simulink model "Copy_of_TenMutantsTemplate"  (R2017b)
settings: Solver=ode3  StartTime=0.0  StopTime=inf  FixedStep=ts  RelTol=0.01  EnableMultiTasking=on
InitFcn:
  | ts=0.0005
  | %ts=100e-6;
StartFcn:
  | close all
StopFcn:
  | % Speed Torque Characterstic
  | 
  | 
  | %figure('Units','pixels', ...
  | %'Color',[1 1 1], ...
  | %'Name','Speed Torque Characterstic',...
  | %'NumberTitle','off',...
  | %'Position',[400 50 470 300], ...
  | %'ToolBar','none');
  | 
  | 
  | 
  | %plot(N_pi,Te_pi)
  | %title('Speed Torque Characterstic')
  | %xlabel('Speed [ RPM ]')
  | %ylabel('Electromagnetic Te_pi [ Nm ] ')
  | %grid on
  | %clear p4 p7 param5 param6 param8 parametres visible voltage
  | 
  | 
  | %clc
values from neighbouring files (symbols this model uses):
  TestOrder = [i]    [ExecuteTestSuite.m]    (also in mutants.m)
undefined symbols (not defined in the file or in its folder): emergency_button2, emergency_buttons, tc_simul, tc_size, temperature, trans1, trans2, trans3, trans4
libraries: simulink x44, powerlib_extras x11
(part 1 of 5)
CloseFcn:
  | close all
settings Model: Creator=srikanth  LastModifiedBy=aarrieta
settings DataIOCC: SaveFormat=Array  SignalLoggingSaveFormat=ModelDataLogs  SaveOutput=off  SaveTime=off  TimeSaveName=t  OutputSaveName=speed,torque,ref
settings OptimizationCC: ExpressionDepthLimit=2147483647  LifeSpan=inf
settings DebuggingCC: UnderspecifiedInitializationDetection=Classic  MergeDetectMultiDrivingBlocksExec=none  ParameterPrecisionLossMsg=none  FcnCallInpInsideContextMsg=warning  StateNameClashWarn=warning  SFUnexpectedBacktrackingDiag=warning  SFNoUnconditionalDefaultTransitionDiag=warning  SFExecutionAtInitializationDiag=none
settings HardwareCC: ProdBitPerPointer=32  ProdBitPerSizeT=32  ProdBitPerPtrDiffT=32  ProdLargestAtomicFloat=None  ProdIntDivRoundTo=Undefined  ProdEndianess=Unspecified  ProdWordSize=32  ProdHWDeviceType=32-bit Generic
settings ModelReferenceCC: PropagateSignalLabelsOutOfModel=off
settings CodeAppCC: StateflowObjectComments=on
settings GRTTargetCC: TargetLangStandard=C89/C90 (ANSI)  GeneratePreprocessorConditionals=Disable all  CombineOutputUpdateFcns=off  GRTInterface=on
settings ConfigComp: CovMetricSettings=dw  CovHtmlReporting=on  CovSaveCumulativeToWorkspaceVar=on  CovSaveSingleToWorkspaceVar=on  CovExternalEMLEnable=off

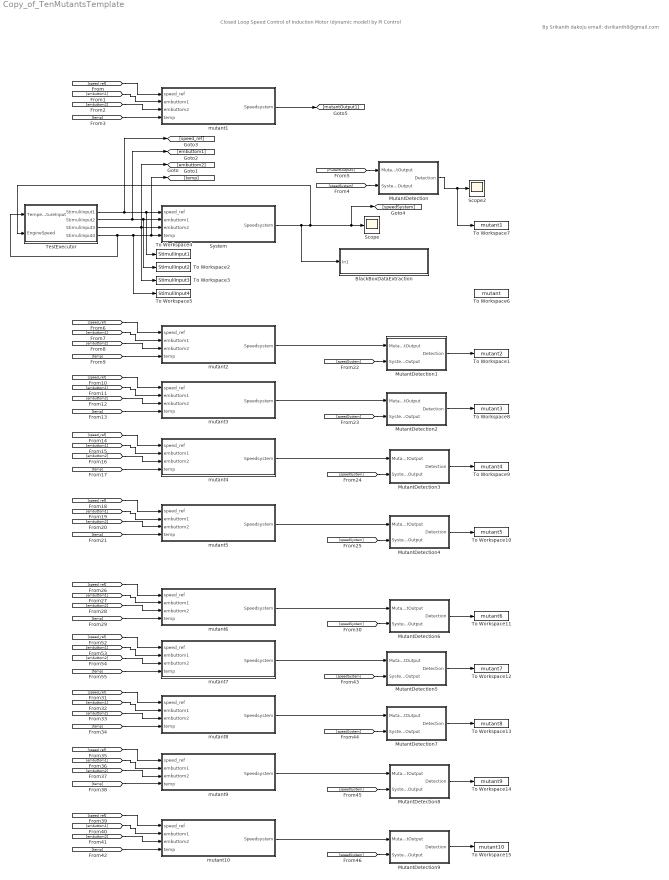
== system Copy_of_TenMutantsTemplate ==
  note: Closed Loop Speed Control of Induction Motor (dynamic model) by PI Control
  note: By
      | Srikanth dakoju
      | email: dsrikanth8@gmail.com
  BlackBoxDataExtraction : Subsystem
  MutantDetection : Subsystem
  MutantDetection1 : Subsystem
  MutantDetection2 : Subsystem
  MutantDetection3 : Subsystem
  MutantDetection4 : Subsystem
  MutantDetection5 : Subsystem
  MutantDetection6 : Subsystem
  MutantDetection7 : Subsystem
  MutantDetection8 : Subsystem
  MutantDetection9 : Subsystem
  Scope : Scope
  Scope2 : Scope
  System : Subsystem
  TestExecutor : Subsystem
  To Workspace1 : ToWorkspace  VariableName=mutant2  SampleTime=-1
  To Workspace10 : ToWorkspace  VariableName=mutant5  SampleTime=-1
  To Workspace11 : ToWorkspace  VariableName=mutant6  SampleTime=-1
  To Workspace12 : ToWorkspace  VariableName=mutant7  SampleTime=-1
  To Workspace13 : ToWorkspace  VariableName=mutant8  SampleTime=-1
  To Workspace14 : ToWorkspace  VariableName=mutant9  SampleTime=-1
  To Workspace15 : ToWorkspace  VariableName=mutant10  SampleTime=-1
  To Workspace2 : ToWorkspace  VariableName=StimuliInput2  SampleTime=-1
  To Workspace3 : ToWorkspace  VariableName=StimuliInput3  SampleTime=-1
  To Workspace4 : ToWorkspace  VariableName=StimuliInput1  SampleTime=-1
  To Workspace5 : ToWorkspace  VariableName=StimuliInput4  SampleTime=-1
  To Workspace6 : ToWorkspace  VariableName=mutant  SampleTime=-1
  To Workspace7 : ToWorkspace  VariableName=mutant1  SampleTime=-1
  To Workspace8 : ToWorkspace  VariableName=mutant3  SampleTime=-1
  To Workspace9 : ToWorkspace  VariableName=mutant4  SampleTime=-1
  mutant1 : Subsystem
  mutant10 : Subsystem
  mutant2 : Subsystem
  mutant3 : Subsystem
  mutant4 : Subsystem
  mutant5 : Subsystem
  mutant6 : Subsystem
  mutant7 : Subsystem
  mutant8 : Subsystem
  mutant9 : Subsystem
  wires:
  TestExecutor/2(StimuliInput2) -> [embuttom1], To Workspace2/1, System/2(embuttom1)
  TestExecutor/3(StimuliInput3) -> [embuttom2], To Workspace3/1, System/3(embuttom2)
  TestExecutor/4(StimuliInput4) -> TestExecutor/1(TemperatureInput), To Workspace5/1, [temp], System/4(temp)
  System/1(Speedsystem) -> BlackBoxDataExtraction/1(In1), TestExecutor/2(EngineSpeed), [speedSystem], Scope/1
  TestExecutor/1(StimuliInput1) -> [speed_ref], To Workspace4/1, System/1(speed_ref)
  mutant1/1(Speedsystem) -> [mutantOutput1]
  MutantDetection/1(Detection) -> To Workspace7/1, Scope2/1
  [temp] -> mutant1/4(temp)
  [embuttom2] -> mutant1/3(embuttom2)
  [embuttom1] -> mutant1/2(embuttom1)
  [speed_ref] -> mutant1/1(speed_ref)
  [speedSystem] -> MutantDetection/2(SystemOutput)
  [mutantOutput1] -> MutantDetection/1(MutantOutput)
  [speed_ref] -> mutant2/1(speed_ref)
  [embuttom1] -> mutant2/2(embuttom1)
  [embuttom2] -> mutant2/3(embuttom2)
  [temp] -> mutant2/4(temp)
  mutant3/1(Speedsystem) -> MutantDetection2/1(MutantOutput)
  [temp] -> mutant3/4(temp)
  [embuttom2] -> mutant3/3(embuttom2)
  [embuttom1] -> mutant3/2(embuttom1)
  [speed_ref] -> mutant3/1(speed_ref)
  [speed_ref] -> mutant4/1(speed_ref)
  [embuttom1] -> mutant4/2(embuttom1)
  [embuttom2] -> mutant4/3(embuttom2)
  [temp] -> mutant4/4(temp)
  mutant5/1(Speedsystem) -> MutantDetection4/1(MutantOutput)
  [temp] -> mutant5/4(temp)
  [embuttom2] -> mutant5/3(embuttom2)
  [embuttom1] -> mutant5/2(embuttom1)
  [speed_ref] -> mutant5/1(speed_ref)
  mutant2/1(Speedsystem) -> MutantDetection1/1(MutantOutput)
  [speedSystem] -> MutantDetection1/2(SystemOutput)
  MutantDetection1/1(Detection) -> To Workspace1/1
  [speedSystem] -> MutantDetection2/2(SystemOutput)
  [speedSystem] -> MutantDetection3/2(SystemOutput)
  mutant4/1(Speedsystem) -> MutantDetection3/1(MutantOutput)
  [speedSystem] -> MutantDetection4/2(SystemOutput)
  MutantDetection4/1(Detection) -> To Workspace10/1
  MutantDetection3/1(Detection) -> To Workspace9/1
  MutantDetection2/1(Detection) -> To Workspace8/1
  MutantDetection6/1(Detection) -> To Workspace11/1
  [speedSystem] -> MutantDetection6/2(SystemOutput)
  [speed_ref] -> mutant6/1(speed_ref)
  [embuttom1] -> mutant6/2(embuttom1)
  [embuttom2] -> mutant6/3(embuttom2)
  [temp] -> mutant6/4(temp)
  mutant6/1(Speedsystem) -> MutantDetection6/1(MutantOutput)
  mutant7/1(Speedsystem) -> MutantDetection5/1(MutantOutput)
  [embuttom1] -> mutant8/2(embuttom1)
  [speed_ref] -> mutant8/1(speed_ref)
  [embuttom2] -> mutant8/3(embuttom2)
  [temp] -> mutant8/4(temp)
  [embuttom1] -> mutant7/2(embuttom1)
  [speed_ref] -> mutant7/1(speed_ref)
  [embuttom2] -> mutant7/3(embuttom2)
  [embuttom2] -> mutant10/3(embuttom2)
  [temp] -> mutant10/4(temp)
  [speed_ref] -> mutant10/1(speed_ref)
  mutant10/1(Speedsystem) -> MutantDetection9/1(MutantOutput)
  mutant8/1(Speedsystem) -> MutantDetection7/1(MutantOutput)
  [speedSystem] -> MutantDetection9/2(SystemOutput)
  [speed_ref] -> mutant9/1(speed_ref)
  [embuttom2] -> mutant9/3(embuttom2)
  [speedSystem] -> MutantDetection7/2(SystemOutput)
  [embuttom1] -> mutant10/2(embuttom1)
  MutantDetection5/1(Detection) -> To Workspace12/1
  mutant9/1(Speedsystem) -> MutantDetection8/1(MutantOutput)
  [temp] -> mutant9/4(temp)
  [embuttom1] -> mutant9/2(embuttom1)
  [speedSystem] -> MutantDetection5/2(SystemOutput)
  [speedSystem] -> MutantDetection8/2(SystemOutput)
  [temp] -> mutant7/4(temp)
  MutantDetection8/1(Detection) -> To Workspace14/1
  MutantDetection7/1(Detection) -> To Workspace13/1
  MutantDetection9/1(Detection) -> To Workspace15/1

== system Copy_of_TenMutantsTemplate/BlackBoxDataExtraction ==
  In1 : Inport
  Abs2 : Abs
  Abs3 : Abs
  Add1 : Sum  Inputs=+-
  Add2 : Sum  Inputs=+-
  Clock : Clock
  Infinite1 : Scope
  Memory{3..7} (5 alike) : Memory
  MinMax2 : MinMax  Function=max  Inputs=2
  MinMax3 : MinMax  Function=max  Inputs=2
  MinMax4 : MinMax  Function=max  Inputs=2
  MinMax5 : MinMax  Inputs=2
  Rate Transition1 : RateTransition
  To Workspace1 : ToWorkspace  VariableName=MaxMin1  SampleTime=-1
  To Workspace10 : ToWorkspace  VariableName=Output1  SampleTime=-1
  To Workspace13 : ToWorkspace  VariableName=Derivative1  SampleTime=-1
  To Workspace14 : ToWorkspace  VariableName=Infinite1  SampleTime=-1
  To Workspace2 : ToWorkspace  VariableName=time  SampleTime=-1
  derive1 : Scope
  throt : Scope
  wires:
  MinMax3/1 -> Memory4/1, To Workspace14/1, Infinite1/1
  Memory3/1 -> MinMax2/2
  MinMax5/1 -> Add2/2, Memory7/1
  Memory7/1 -> MinMax5/2
  Memory4/1 -> MinMax3/2
  MinMax2/1 -> To Workspace13/1, derive1/1, Memory3/1
  MinMax4/1 -> Add2/1, Memory6/1
  Rate Transition1/1 -> MinMax4/1, MinMax5/1, Abs3/1, Add1/1, Memory5/1
  Memory5/1 -> Add1/2
  Abs2/1 -> MinMax2/1
  Abs3/1 -> MinMax3/1
  Add1/1 -> Abs2/1
  Memory6/1 -> MinMax4/2
  Add2/1 -> To Workspace1/1
  In1/1 -> throt/1, Rate Transition1/1, To Workspace10/1
  Clock/1 -> To Workspace2/1

== system Copy_of_TenMutantsTemplate/MutantDetection ==
  MutantOutput : Inport
  SystemOutput : Inport  Port=2
  Logical Operator : Logic  Operator=NOT  AllPortsSameDT=off  OutDataTypeStr=boolean
  Memory : Memory  InitialCondition=1
  MinMax : MinMax  Inputs=2
  Relational Operator : RelationalOperator  Operator===  OutDataTypeStr=boolean  RndMeth=Simplest
  Detection : Outport
  wires:
  Memory/1 -> MinMax/2
  MinMax/1 -> Logical Operator/1, Memory/1
  MutantOutput/1 -> Relational Operator/1
  SystemOutput/1 -> Relational Operator/2
  Relational Operator/1 -> MinMax/1
  Logical Operator/1 -> Detection/1

== system Copy_of_TenMutantsTemplate/MutantDetection1 ==
  MutantOutput : Inport
  SystemOutput : Inport  Port=2
  Logical Operator : Logic  Operator=NOT  AllPortsSameDT=off  OutDataTypeStr=boolean
  Memory : Memory  InitialCondition=1
  MinMax : MinMax  Inputs=2
  Relational Operator : RelationalOperator  Operator===  OutDataTypeStr=boolean  RndMeth=Simplest
  Detection : Outport
  wires:
  Logical Operator/1 -> Detection/1
  Relational Operator/1 -> MinMax/1
  SystemOutput/1 -> Relational Operator/2
  MutantOutput/1 -> Relational Operator/1
  MinMax/1 -> Memory/1, Logical Operator/1
  Memory/1 -> MinMax/2

== system Copy_of_TenMutantsTemplate/MutantDetection2 ==
  MutantOutput : Inport
  SystemOutput : Inport  Port=2
  Logical Operator : Logic  Operator=NOT  AllPortsSameDT=off  OutDataTypeStr=boolean
  Memory : Memory  InitialCondition=1
  MinMax : MinMax  Inputs=2
  Relational Operator : RelationalOperator  Operator===  OutDataTypeStr=boolean  RndMeth=Simplest
  Detection : Outport
  wires:
  Memory/1 -> MinMax/2
  MinMax/1 -> Logical Operator/1, Memory/1
  MutantOutput/1 -> Relational Operator/1
  SystemOutput/1 -> Relational Operator/2
  Relational Operator/1 -> MinMax/1
  Logical Operator/1 -> Detection/1

== system Copy_of_TenMutantsTemplate/MutantDetection3 ==
  MutantOutput : Inport
  SystemOutput : Inport  Port=2
  Logical Operator : Logic  Operator=NOT  AllPortsSameDT=off  OutDataTypeStr=boolean
  Memory : Memory  InitialCondition=1
  MinMax : MinMax  Inputs=2
  Relational Operator : RelationalOperator  Operator===  OutDataTypeStr=boolean  RndMeth=Simplest
  Detection : Outport
  wires:
  Logical Operator/1 -> Detection/1
  Relational Operator/1 -> MinMax/1
  SystemOutput/1 -> Relational Operator/2
  MutantOutput/1 -> Relational Operator/1
  MinMax/1 -> Memory/1, Logical Operator/1
  Memory/1 -> MinMax/2

== system Copy_of_TenMutantsTemplate/MutantDetection4 ==
  MutantOutput : Inport
  SystemOutput : Inport  Port=2
  Logical Operator : Logic  Operator=NOT  AllPortsSameDT=off  OutDataTypeStr=boolean
  Memory : Memory  InitialCondition=1
  MinMax : MinMax  Inputs=2
  Relational Operator : RelationalOperator  Operator===  OutDataTypeStr=boolean  RndMeth=Simplest
  Detection : Outport
  wires:
  Memory/1 -> MinMax/2
  MinMax/1 -> Logical Operator/1, Memory/1
  MutantOutput/1 -> Relational Operator/1
  SystemOutput/1 -> Relational Operator/2
  Relational Operator/1 -> MinMax/1
  Logical Operator/1 -> Detection/1

== system Copy_of_TenMutantsTemplate/MutantDetection5 ==
  MutantOutput : Inport
  SystemOutput : Inport  Port=2
  Logical Operator : Logic  Operator=NOT  AllPortsSameDT=off  OutDataTypeStr=boolean
  Memory : Memory  InitialCondition=1
  MinMax : MinMax  Inputs=2
  Relational Operator : RelationalOperator  Operator===  OutDataTypeStr=boolean  RndMeth=Simplest
  Detection : Outport
  wires:
  Logical Operator/1 -> Detection/1
  Relational Operator/1 -> MinMax/1
  SystemOutput/1 -> Relational Operator/2
  MutantOutput/1 -> Relational Operator/1
  MinMax/1 -> Memory/1, Logical Operator/1
  Memory/1 -> MinMax/2

== system Copy_of_TenMutantsTemplate/MutantDetection6 ==
  MutantOutput : Inport
  SystemOutput : Inport  Port=2
  Logical Operator : Logic  Operator=NOT  AllPortsSameDT=off  OutDataTypeStr=boolean
  Memory : Memory  InitialCondition=1
  MinMax : MinMax  Inputs=2
  Relational Operator : RelationalOperator  Operator===  OutDataTypeStr=boolean  RndMeth=Simplest
  Detection : Outport
  wires:
  Logical Operator/1 -> Detection/1
  Relational Operator/1 -> MinMax/1
  SystemOutput/1 -> Relational Operator/2
  MutantOutput/1 -> Relational Operator/1
  MinMax/1 -> Memory/1, Logical Operator/1
  Memory/1 -> MinMax/2

== system Copy_of_TenMutantsTemplate/MutantDetection7 ==
  MutantOutput : Inport
  SystemOutput : Inport  Port=2
  Logical Operator : Logic  Operator=NOT  AllPortsSameDT=off  OutDataTypeStr=boolean
  Memory : Memory  InitialCondition=1
  MinMax : MinMax  Inputs=2
  Relational Operator : RelationalOperator  Operator===  OutDataTypeStr=boolean  RndMeth=Simplest
  Detection : Outport
  wires:
  Memory/1 -> MinMax/2
  MinMax/1 -> Logical Operator/1, Memory/1
  MutantOutput/1 -> Relational Operator/1
  SystemOutput/1 -> Relational Operator/2
  Relational Operator/1 -> MinMax/1
  Logical Operator/1 -> Detection/1

== system Copy_of_TenMutantsTemplate/MutantDetection8 ==
  MutantOutput : Inport
  SystemOutput : Inport  Port=2
  Logical Operator : Logic  Operator=NOT  AllPortsSameDT=off  OutDataTypeStr=boolean
  Memory : Memory  InitialCondition=1
  MinMax : MinMax  Inputs=2
  Relational Operator : RelationalOperator  Operator===  OutDataTypeStr=boolean  RndMeth=Simplest
  Detection : Outport
  wires:
  Logical Operator/1 -> Detection/1
  Relational Operator/1 -> MinMax/1
  SystemOutput/1 -> Relational Operator/2
  MutantOutput/1 -> Relational Operator/1
  MinMax/1 -> Memory/1, Logical Operator/1
  Memory/1 -> MinMax/2

== system Copy_of_TenMutantsTemplate/MutantDetection9 ==
  MutantOutput : Inport
  SystemOutput : Inport  Port=2
  Logical Operator : Logic  Operator=NOT  AllPortsSameDT=off  OutDataTypeStr=boolean
  Memory : Memory  InitialCondition=1
  MinMax : MinMax  Inputs=2
  Relational Operator : RelationalOperator  Operator===  OutDataTypeStr=boolean  RndMeth=Simplest
  Detection : Outport
  wires:
  Memory/1 -> MinMax/2
  MinMax/1 -> Logical Operator/1, Memory/1
  MutantOutput/1 -> Relational Operator/1
  SystemOutput/1 -> Relational Operator/2
  Relational Operator/1 -> MinMax/1
  Logical Operator/1 -> Detection/1

== system Copy_of_TenMutantsTemplate/System ==
  note: ctrl+U to look under mask
  speed_ref : Inport
  embuttom1 : Inport  Port=2
  embuttom2 : Inport  Port=3
  temp : Inport  Port=4
  "1 HP , 220 V Induction Motor" : Subsystem  mask(Induction Motor: By SRIKANTH D){Rs=10.1, Ls=(15.81+245.8954)/(2*pi*50), Rr=9.8546, Lr=(15.81+245.8954)/(2*pi*50), Lm=(245.8954)/(2*pi*50), J=0.0088, P=4}
      mask prompts: Rs "Stator Resistance  Rs [ohms] :"; Ls "Stator Inductance Ls [Hendry] :"; Rr "Rotor Resistance Rr [ohms] :"; Lr "Rotor Inductance Lr [Hendry] :"; Lm "Mutual Inductance Lm [Hendry] :"; J "Rotor Inertia J [Kg-m2] :"; P "Number of Poles p :"
      mask help: Dynamic Modelling of Induction by using Mathematic Equations
      mask Display: fprintf('Induction\nMotor')
  Data Acquision : Subsystem
  PI Control1 : Subsystem
      mask Display: fprintf('PI\Control')
  Selector : Selector  InputPortWidth=2  IndexOptions=Index vector (dialog)  Indices=[1]  OutputSizes=1
  Subsystem : Subsystem
  Terminator : Terminator
  Terminator1 : Terminator
  VSI : Subsystem
      mask init:
      | Vdc=220;
      mask Display: fprintf('Vdc = 220 V ')
  torque : Step  Time=2  After=0  SampleTime=0
  Speedsystem : Outport
  wires:
  temp/1 -> Subsystem/4(Temperature)
  "1 HP , 220 V Induction Motor"/1(m) -> Data Acquision/1(m)
  VSI/2(Vb) -> "1 HP , 220 V Induction Motor"/3(V_b)
  Data Acquision/3(wm) -> Selector/1  "Speed( rpm)"
  Data Acquision/4(wm1) -> Speedsystem/1
  embuttom2/1 -> Subsystem/3(EmergButton2)
  embuttom1/1 -> Subsystem/2(EmergButton1)
  speed_ref/1 -> Subsystem/1(Speed)
  Data Acquision/2(Te(Nm)) -> Terminator/1  "Torque Te(Nm)"
  Subsystem/1("MotorSpeed ") -> Data Acquision/2(speed), PI Control1/1(N*)
  PI Control1/1(Freq*) -> VSI/1(Freq)
  torque/1 -> "1 HP , 220 V Induction Motor"/1(tau)
  Selector/1 -> PI Control1/2(N)
  VSI/1(Va) -> "1 HP , 220 V Induction Motor"/2(V_a)
  VSI/3(Vc) -> "1 HP , 220 V Induction Motor"/4(V_c)
  Data Acquision/1(is_a) -> Terminator1/1

== system Copy_of_TenMutantsTemplate/TestExecutor ==
  TemperatureInput : Inport
  EngineSpeed : Inport  Port=2
  Constant : Constant  Value=TestOrder
  Constant10 : Constant  Value=trans4
  Constant3 : Constant  Value=tc_simul
  Constant4 : Constant  Value=tc_size
  Constant7 : Constant  Value=trans1
  Constant8 : Constant  Value=trans2
  Constant9 : Constant  Value=trans3
  MATLAB Function : MATLAB Function  TreatAsAtomicUnit=on
  MATLAB Function1 : MATLAB Function  TreatAsAtomicUnit=on
  Memory{,1..3} (4 alike) : Memory  InitialCondition=1
  Scope : Scope
  Scope1 : Scope
  Stop Simulation : Stop
  StimuliInput1 : Outport
  StimuliInput2 : Outport  Port=2
  StimuliInput3 : Outport  Port=3
  StimuliInput4 : Outport  Port=4
  wires:
  Memory3/1 -> MATLAB Function1/7(v_engine)
  Memory2/1 -> MATLAB Function1/8(temp)
  MATLAB Function1/5(simulation_stop) -> Stop Simulation/1
  MATLAB Function1/2(state) -> Scope1/1, MATLAB Function/3(state)
  MATLAB Function1/1(test_case) -> MATLAB Function/2(test_case), Scope/1
  EngineSpeed/1 -> Memory3/1
  Memory1/1 -> MATLAB Function1/9(test_order_id)
  Memory/1 -> MATLAB Function1/10(state_id)
  MATLAB Function1/3(test_order_id1) -> Memory1/1
  MATLAB Function1/4(state_id1) -> Memory/1
  Constant10/1 -> MATLAB Function1/6(trans4)
  Constant9/1 -> MATLAB Function1/5(trans3)
  Constant8/1 -> MATLAB Function1/4(trans2)
  Constant7/1 -> MATLAB Function1/3(trans1)
  Constant4/1 -> MATLAB Function1/2(tc_size)
  Constant/1 -> MATLAB Function1/1(test_order)
  Constant3/1 -> MATLAB Function/1(tc_simul)
  MATLAB Function/4(port_4) -> StimuliInput4/1
  MATLAB Function/3(port_3) -> StimuliInput3/1
  MATLAB Function/2(port_2) -> StimuliInput2/1
  MATLAB Function/1(port_1) -> StimuliInput1/1
  TemperatureInput/1 -> Memory2/1

== system Copy_of_TenMutantsTemplate/mutant1 ==
  note: ctrl+U to look under mask
  speed_ref : Inport
  embuttom1 : Inport  Port=2
  embuttom2 : Inport  Port=3
  temp : Inport  Port=4
  "1 HP , 220 V Induction Motor" : Subsystem  mask(Induction Motor: By SRIKANTH D){Rs=10.1, Ls=(15.81+245.8954)/(2*pi*50), Rr=9.8546, Lr=(15.81+245.8954)/(2*pi*50), Lm=(245.8954)/(2*pi*50), J=0.0088, P=4}
      mask prompts: Rs "Stator Resistance  Rs [ohms] :"; Ls "Stator Inductance Ls [Hendry] :"; Rr "Rotor Resistance Rr [ohms] :"; Lr "Rotor Inductance Lr [Hendry] :"; Lm "Mutual Inductance Lm [Hendry] :"; J "Rotor Inertia J [Kg-m2] :"; P "Number of Poles p :"
      mask help: Dynamic Modelling of Induction by using Mathematic Equations
      mask Display: fprintf('Induction\nMotor')
  Data Acquision : Subsystem
  PI Control1 : Subsystem
      mask Display: fprintf('PI\Control')
  Selector : Selector  InputPortWidth=2  IndexOptions=Index vector (dialog)  Indices=[1]  OutputSizes=1
  Subsystem : Subsystem
  Terminator : Terminator
  Terminator1 : Terminator
  VSI : Subsystem
      mask init:
      | Vdc=220;
      mask Display: fprintf('Vdc = 220 V ')
  torque : Step  Time=2  After=0  SampleTime=0
  Speedsystem : Outport
  wires:
  Data Acquision/1(is_a) -> Terminator1/1
  VSI/3(Vc) -> "1 HP , 220 V Induction Motor"/4(V_c)
  VSI/1(Va) -> "1 HP , 220 V Induction Motor"/2(V_a)
  Selector/1 -> PI Control1/2(N)
  torque/1 -> "1 HP , 220 V Induction Motor"/1(tau)
  PI Control1/1(Freq*) -> VSI/1(Freq)
  Subsystem/1("MotorSpeed ") -> PI Control1/1(N*), Data Acquision/2(speed)
  Data Acquision/2(Te(Nm)) -> Terminator/1  "Torque Te(Nm)"
  speed_ref/1 -> Subsystem/1(Speed)
  embuttom1/1 -> Subsystem/2(EmergButton1)
  embuttom2/1 -> Subsystem/3(EmergButton2)
  Data Acquision/4(wm1) -> Speedsystem/1
  Data Acquision/3(wm) -> Selector/1  "Speed( rpm)"
  VSI/2(Vb) -> "1 HP , 220 V Induction Motor"/3(V_b)
  "1 HP , 220 V Induction Motor"/1(m) -> Data Acquision/1(m)
  temp/1 -> Subsystem/4(Temperature)

== system Copy_of_TenMutantsTemplate/mutant10 ==
  note: ctrl+U to look under mask
  speed_ref : Inport
  embuttom1 : Inport  Port=2
  embuttom2 : Inport  Port=3
  temp : Inport  Port=4
  "1 HP , 220 V Induction Motor" : Subsystem  mask(Induction Motor: By SRIKANTH D){Rs=10.1, Ls=(15.81+245.8954)/(2*pi*50), Rr=9.8546, Lr=(15.81+245.8954)/(2*pi*50), Lm=(245.8954)/(2*pi*50), J=0.0088, P=4}
      mask prompts: Rs "Stator Resistance  Rs [ohms] :"; Ls "Stator Inductance Ls [Hendry] :"; Rr "Rotor Resistance Rr [ohms] :"; Lr "Rotor Inductance Lr [Hendry] :"; Lm "Mutual Inductance Lm [Hendry] :"; J "Rotor Inertia J [Kg-m2] :"; P "Number of Poles p :"
      mask help: Dynamic Modelling of Induction by using Mathematic Equations
      mask Display: fprintf('Induction\nMotor')
  Data Acquision : Subsystem
  PI Control1 : Subsystem
      mask Display: fprintf('PI\Control')
  Selector : Selector  InputPortWidth=2  IndexOptions=Index vector (dialog)  Indices=[1]  OutputSizes=1
  Subsystem : Subsystem
  Terminator : Terminator
  Terminator1 : Terminator
  VSI : Subsystem
      mask init:
      | Vdc=220;
      mask Display: fprintf('Vdc = 220 V ')
  torque : Step  Time=2  After=0  SampleTime=0
  Speedsystem : Outport
  wires:
  Data Acquision/1(is_a) -> Terminator1/1
  VSI/3(Vc) -> "1 HP , 220 V Induction Motor"/4(V_c)
  VSI/1(Va) -> "1 HP , 220 V Induction Motor"/2(V_a)
  Selector/1 -> PI Control1/2(N)
  torque/1 -> "1 HP , 220 V Induction Motor"/1(tau)
  PI Control1/1(Freq*) -> VSI/1(Freq)
  Subsystem/1("MotorSpeed ") -> PI Control1/1(N*), Data Acquision/2(speed)
  Data Acquision/2(Te(Nm)) -> Terminator/1  "Torque Te(Nm)"
  speed_ref/1 -> Subsystem/1(Speed)
  embuttom1/1 -> Subsystem/2(EmergButton1)
  embuttom2/1 -> Subsystem/3(EmergButton2)
  Data Acquision/4(wm1) -> Speedsystem/1
  Data Acquision/3(wm) -> Selector/1  "Speed( rpm)"
  VSI/2(Vb) -> "1 HP , 220 V Induction Motor"/3(V_b)
  "1 HP , 220 V Induction Motor"/1(m) -> Data Acquision/1(m)
  temp/1 -> Subsystem/4(Temperature)

== system Copy_of_TenMutantsTemplate/mutant2 ==
  note: ctrl+U to look under mask
  speed_ref : Inport
  embuttom1 : Inport  Port=2
  embuttom2 : Inport  Port=3
  temp : Inport  Port=4
  "1 HP , 220 V Induction Motor" : Subsystem  mask(Induction Motor: By SRIKANTH D){Rs=10.1, Ls=(15.81+245.8954)/(2*pi*50), Rr=9.8546, Lr=(15.81+245.8954)/(2*pi*50), Lm=(245.8954)/(2*pi*50), J=0.0088, P=4}
      mask prompts: Rs "Stator Resistance  Rs [ohms] :"; Ls "Stator Inductance Ls [Hendry] :"; Rr "Rotor Resistance Rr [ohms] :"; Lr "Rotor Inductance Lr [Hendry] :"; Lm "Mutual Inductance Lm [Hendry] :"; J "Rotor Inertia J [Kg-m2] :"; P "Number of Poles p :"
      mask help: Dynamic Modelling of Induction by using Mathematic Equations
      mask Display: fprintf('Induction\nMotor')
  Data Acquision : Subsystem
  PI Control1 : Subsystem
      mask Display: fprintf('PI\Control')
  Selector : Selector  InputPortWidth=2  IndexOptions=Index vector (dialog)  Indices=[1]  OutputSizes=1
  Subsystem : Subsystem
  Terminator : Terminator
  Terminator1 : Terminator
  VSI : Subsystem
      mask init:
      | Vdc=220;
      mask Display: fprintf('Vdc = 220 V ')
  torque : Step  Time=2  After=0  SampleTime=0
  Speedsystem : Outport
  wires:
  temp/1 -> Subsystem/4(Temperature)
  "1 HP , 220 V Induction Motor"/1(m) -> Data Acquision/1(m)
  VSI/2(Vb) -> "1 HP , 220 V Induction Motor"/3(V_b)
  Data Acquision/3(wm) -> Selector/1  "Speed( rpm)"
  Data Acquision/4(wm1) -> Speedsystem/1
  embuttom2/1 -> Subsystem/3(EmergButton2)
  embuttom1/1 -> Subsystem/2(EmergButton1)
  speed_ref/1 -> Subsystem/1(Speed)
  Data Acquision/2(Te(Nm)) -> Terminator/1  "Torque Te(Nm)"
  Subsystem/1("MotorSpeed ") -> Data Acquision/2(speed), PI Control1/1(N*)
  PI Control1/1(Freq*) -> VSI/1(Freq)
  torque/1 -> "1 HP , 220 V Induction Motor"/1(tau)
  Selector/1 -> PI Control1/2(N)
  VSI/1(Va) -> "1 HP , 220 V Induction Motor"/2(V_a)
  VSI/3(Vc) -> "1 HP , 220 V Induction Motor"/4(V_c)
  Data Acquision/1(is_a) -> Terminator1/1

== system Copy_of_TenMutantsTemplate/mutant3 ==
  note: ctrl+U to look under mask
  speed_ref : Inport
  embuttom1 : Inport  Port=2
  embuttom2 : Inport  Port=3
  temp : Inport  Port=4
  "1 HP , 220 V Induction Motor" : Subsystem  mask(Induction Motor: By SRIKANTH D){Rs=10.1, Ls=(15.81+245.8954)/(2*pi*50), Rr=9.8546, Lr=(15.81+245.8954)/(2*pi*50), Lm=(245.8954)/(2*pi*50), J=0.0088, P=4}
      mask prompts: Rs "Stator Resistance  Rs [ohms] :"; Ls "Stator Inductance Ls [Hendry] :"; Rr "Rotor Resistance Rr [ohms] :"; Lr "Rotor Inductance Lr [Hendry] :"; Lm "Mutual Inductance Lm [Hendry] :"; J "Rotor Inertia J [Kg-m2] :"; P "Number of Poles p :"
      mask help: Dynamic Modelling of Induction by using Mathematic Equations
      mask Display: fprintf('Induction\nMotor')
  Data Acquision : Subsystem
  PI Control1 : Subsystem
      mask Display: fprintf('PI\Control')
  Selector : Selector  InputPortWidth=2  IndexOptions=Index vector (dialog)  Indices=[1]  OutputSizes=1
  Subsystem : Subsystem
  Terminator : Terminator
  Terminator1 : Terminator
  VSI : Subsystem
      mask init:
      | Vdc=220;
      mask Display: fprintf('Vdc = 220 V ')
  torque : Step  Time=2  After=0  SampleTime=0
  Speedsystem : Outport
  wires:
  Data Acquision/1(is_a) -> Terminator1/1
  VSI/3(Vc) -> "1 HP , 220 V Induction Motor"/4(V_c)
  VSI/1(Va) -> "1 HP , 220 V Induction Motor"/2(V_a)
  Selector/1 -> PI Control1/2(N)
  torque/1 -> "1 HP , 220 V Induction Motor"/1(tau)
  PI Control1/1(Freq*) -> VSI/1(Freq)
  Subsystem/1("MotorSpeed ") -> PI Control1/1(N*), Data Acquision/2(speed)
  Data Acquision/2(Te(Nm)) -> Terminator/1  "Torque Te(Nm)"
  speed_ref/1 -> Subsystem/1(Speed)
  embuttom1/1 -> Subsystem/2(EmergButton1)
  embuttom2/1 -> Subsystem/3(EmergButton2)
  Data Acquision/4(wm1) -> Speedsystem/1
  Data Acquision/3(wm) -> Selector/1  "Speed( rpm)"
  VSI/2(Vb) -> "1 HP , 220 V Induction Motor"/3(V_b)
  "1 HP , 220 V Induction Motor"/1(m) -> Data Acquision/1(m)
  temp/1 -> Subsystem/4(Temperature)

== system Copy_of_TenMutantsTemplate/mutant4 ==
  note: ctrl+U to look under mask
  speed_ref : Inport
  embuttom1 : Inport  Port=2
  embuttom2 : Inport  Port=3
  temp : Inport  Port=4
  "1 HP , 220 V Induction Motor" : Subsystem  mask(Induction Motor: By SRIKANTH D){Rs=10.1, Ls=(15.81+245.8954)/(2*pi*50), Rr=9.8546, Lr=(15.81+245.8954)/(2*pi*50), Lm=(245.8954)/(2*pi*50), J=0.0088, P=4}
      mask prompts: Rs "Stator Resistance  Rs [ohms] :"; Ls "Stator Inductance Ls [Hendry] :"; Rr "Rotor Resistance Rr [ohms] :"; Lr "Rotor Inductance Lr [Hendry] :"; Lm "Mutual Inductance Lm [Hendry] :"; J "Rotor Inertia J [Kg-m2] :"; P "Number of Poles p :"
      mask help: Dynamic Modelling of Induction by using Mathematic Equations
      mask Display: fprintf('Induction\nMotor')
  Data Acquision : Subsystem
  PI Control1 : Subsystem
      mask Display: fprintf('PI\Control')
  Selector : Selector  InputPortWidth=2  IndexOptions=Index vector (dialog)  Indices=[1]  OutputSizes=1
  Subsystem : Subsystem
  Terminator : Terminator
  Terminator1 : Terminator
  VSI : Subsystem
      mask init:
      | Vdc=220;
      mask Display: fprintf('Vdc = 220 V ')
  torque : Step  Time=2  After=0  SampleTime=0
  Speedsystem : Outport
  wires:
  temp/1 -> Subsystem/4(Temperature)
  "1 HP , 220 V Induction Motor"/1(m) -> Data Acquision/1(m)
  VSI/2(Vb) -> "1 HP , 220 V Induction Motor"/3(V_b)
  Data Acquision/3(wm) -> Selector/1  "Speed( rpm)"
  Data Acquision/4(wm1) -> Speedsystem/1
  embuttom2/1 -> Subsystem/3(EmergButton2)
  embuttom1/1 -> Subsystem/2(EmergButton1)
  speed_ref/1 -> Subsystem/1(Speed)
  Data Acquision/2(Te(Nm)) -> Terminator/1  "Torque Te(Nm)"
  Subsystem/1("MotorSpeed ") -> Data Acquision/2(speed), PI Control1/1(N*)
  PI Control1/1(Freq*) -> VSI/1(Freq)
  torque/1 -> "1 HP , 220 V Induction Motor"/1(tau)
  Selector/1 -> PI Control1/2(N)
  VSI/1(Va) -> "1 HP , 220 V Induction Motor"/2(V_a)
  VSI/3(Vc) -> "1 HP , 220 V Induction Motor"/4(V_c)
  Data Acquision/1(is_a) -> Terminator1/1

== system Copy_of_TenMutantsTemplate/mutant5 ==
  note: ctrl+U to look under mask
  speed_ref : Inport
  embuttom1 : Inport  Port=2
  embuttom2 : Inport  Port=3
  temp : Inport  Port=4
  "1 HP , 220 V Induction Motor" : Subsystem  mask(Induction Motor: By SRIKANTH D){Rs=10.1, Ls=(15.81+245.8954)/(2*pi*50), Rr=9.8546, Lr=(15.81+245.8954)/(2*pi*50), Lm=(245.8954)/(2*pi*50), J=0.0088, P=4}
      mask prompts: Rs "Stator Resistance  Rs [ohms] :"; Ls "Stator Inductance Ls [Hendry] :"; Rr "Rotor Resistance Rr [ohms] :"; Lr "Rotor Inductance Lr [Hendry] :"; Lm "Mutual Inductance Lm [Hendry] :"; J "Rotor Inertia J [Kg-m2] :"; P "Number of Poles p :"
      mask help: Dynamic Modelling of Induction by using Mathematic Equations
      mask Display: fprintf('Induction\nMotor')
  Data Acquision : Subsystem
  PI Control1 : Subsystem
      mask Display: fprintf('PI\Control')
  Selector : Selector  InputPortWidth=2  IndexOptions=Index vector (dialog)  Indices=[1]  OutputSizes=1
  Subsystem : Subsystem
  Terminator : Terminator
  Terminator1 : Terminator
  VSI : Subsystem
      mask init:
      | Vdc=220;
      mask Display: fprintf('Vdc = 220 V ')
  torque : Step  Time=2  After=0  SampleTime=0
  Speedsystem : Outport
  wires:
  Data Acquision/1(is_a) -> Terminator1/1
  VSI/3(Vc) -> "1 HP , 220 V Induction Motor"/4(V_c)
  VSI/1(Va) -> "1 HP , 220 V Induction Motor"/2(V_a)
  Selector/1 -> PI Control1/2(N)
  torque/1 -> "1 HP , 220 V Induction Motor"/1(tau)
  PI Control1/1(Freq*) -> VSI/1(Freq)
  Subsystem/1("MotorSpeed ") -> PI Control1/1(N*), Data Acquision/2(speed)
  Data Acquision/2(Te(Nm)) -> Terminator/1  "Torque Te(Nm)"
  speed_ref/1 -> Subsystem/1(Speed)
  embuttom1/1 -> Subsystem/2(EmergButton1)
  embuttom2/1 -> Subsystem/3(EmergButton2)
  Data Acquision/4(wm1) -> Speedsystem/1
  Data Acquision/3(wm) -> Selector/1  "Speed( rpm)"
  VSI/2(Vb) -> "1 HP , 220 V Induction Motor"/3(V_b)
  "1 HP , 220 V Induction Motor"/1(m) -> Data Acquision/1(m)
  temp/1 -> Subsystem/4(Temperature)

== system Copy_of_TenMutantsTemplate/mutant6 ==
  note: ctrl+U to look under mask
  speed_ref : Inport
  embuttom1 : Inport  Port=2
  embuttom2 : Inport  Port=3
  temp : Inport  Port=4
  "1 HP , 220 V Induction Motor" : Subsystem  mask(Induction Motor: By SRIKANTH D){Rs=10.1, Ls=(15.81+245.8954)/(2*pi*50), Rr=9.8546, Lr=(15.81+245.8954)/(2*pi*50), Lm=(245.8954)/(2*pi*50), J=0.0088, P=4}
      mask prompts: Rs "Stator Resistance  Rs [ohms] :"; Ls "Stator Inductance Ls [Hendry] :"; Rr "Rotor Resistance Rr [ohms] :"; Lr "Rotor Inductance Lr [Hendry] :"; Lm "Mutual Inductance Lm [Hendry] :"; J "Rotor Inertia J [Kg-m2] :"; P "Number of Poles p :"
      mask help: Dynamic Modelling of Induction by using Mathematic Equations
      mask Display: fprintf('Induction\nMotor')
  Data Acquision : Subsystem
  PI Control1 : Subsystem
      mask Display: fprintf('PI\Control')
  Selector : Selector  InputPortWidth=2  IndexOptions=Index vector (dialog)  Indices=[1]  OutputSizes=1
  Subsystem : Subsystem
  Terminator : Terminator
  Terminator1 : Terminator
  VSI : Subsystem
      mask init:
      | Vdc=220;
      mask Display: fprintf('Vdc = 220 V ')
  torque : Step  Time=2  After=0  SampleTime=0
  Speedsystem : Outport
  wires:
  temp/1 -> Subsystem/4(Temperature)
  "1 HP , 220 V Induction Motor"/1(m) -> Data Acquision/1(m)
  VSI/2(Vb) -> "1 HP , 220 V Induction Motor"/3(V_b)
  Data Acquision/3(wm) -> Selector/1  "Speed( rpm)"
  Data Acquision/4(wm1) -> Speedsystem/1
  embuttom2/1 -> Subsystem/3(EmergButton2)
  embuttom1/1 -> Subsystem/2(EmergButton1)
  speed_ref/1 -> Subsystem/1(Speed)
  Data Acquision/2(Te(Nm)) -> Terminator/1  "Torque Te(Nm)"
  Subsystem/1("MotorSpeed ") -> Data Acquision/2(speed), PI Control1/1(N*)
  PI Control1/1(Freq*) -> VSI/1(Freq)
  torque/1 -> "1 HP , 220 V Induction Motor"/1(tau)
  Selector/1 -> PI Control1/2(N)
  VSI/1(Va) -> "1 HP , 220 V Induction Motor"/2(V_a)
  VSI/3(Vc) -> "1 HP , 220 V Induction Motor"/4(V_c)
  Data Acquision/1(is_a) -> Terminator1/1

== system Copy_of_TenMutantsTemplate/mutant7 ==
  note: ctrl+U to look under mask
  speed_ref : Inport
  embuttom1 : Inport  Port=2
  embuttom2 : Inport  Port=3
  temp : Inport  Port=4
  "1 HP , 220 V Induction Motor" : Subsystem  mask(Induction Motor: By SRIKANTH D){Rs=10.1, Ls=(15.81+245.8954)/(2*pi*50), Rr=9.8546, Lr=(15.81+245.8954)/(2*pi*50), Lm=(245.8954)/(2*pi*50), J=0.0088, P=4}
      mask prompts: Rs "Stator Resistance  Rs [ohms] :"; Ls "Stator Inductance Ls [Hendry] :"; Rr "Rotor Resistance Rr [ohms] :"; Lr "Rotor Inductance Lr [Hendry] :"; Lm "Mutual Inductance Lm [Hendry] :"; J "Rotor Inertia J [Kg-m2] :"; P "Number of Poles p :"
      mask help: Dynamic Modelling of Induction by using Mathematic Equations
      mask Display: fprintf('Induction\nMotor')
  Data Acquision : Subsystem
  PI Control1 : Subsystem
      mask Display: fprintf('PI\Control')
  Selector : Selector  InputPortWidth=2  IndexOptions=Index vector (dialog)  Indices=[1]  OutputSizes=1
  Subsystem : Subsystem
  Terminator : Terminator
  Terminator1 : Terminator
  VSI : Subsystem
      mask init:
      | Vdc=220;
      mask Display: fprintf('Vdc = 220 V ')
  torque : Step  Time=2  After=0  SampleTime=0
  Speedsystem : Outport
  wires:
  temp/1 -> Subsystem/4(Temperature)
  "1 HP , 220 V Induction Motor"/1(m) -> Data Acquision/1(m)
  VSI/2(Vb) -> "1 HP , 220 V Induction Motor"/3(V_b)
  Data Acquision/3(wm) -> Selector/1  "Speed( rpm)"
  Data Acquision/4(wm1) -> Speedsystem/1
  embuttom2/1 -> Subsystem/3(EmergButton2)
  embuttom1/1 -> Subsystem/2(EmergButton1)
  speed_ref/1 -> Subsystem/1(Speed)
  Data Acquision/2(Te(Nm)) -> Terminator/1  "Torque Te(Nm)"
  Subsystem/1("MotorSpeed ") -> Data Acquision/2(speed), PI Control1/1(N*)
  PI Control1/1(Freq*) -> VSI/1(Freq)
  torque/1 -> "1 HP , 220 V Induction Motor"/1(tau)
  Selector/1 -> PI Control1/2(N)
  VSI/1(Va) -> "1 HP , 220 V Induction Motor"/2(V_a)
  VSI/3(Vc) -> "1 HP , 220 V Induction Motor"/4(V_c)
  Data Acquision/1(is_a) -> Terminator1/1

== system Copy_of_TenMutantsTemplate/mutant8 ==
  note: ctrl+U to look under mask
  speed_ref : Inport
  embuttom1 : Inport  Port=2
  embuttom2 : Inport  Port=3
  temp : Inport  Port=4
  "1 HP , 220 V Induction Motor" : Subsystem  mask(Induction Motor: By SRIKANTH D){Rs=10.1, Ls=(15.81+245.8954)/(2*pi*50), Rr=9.8546, Lr=(15.81+245.8954)/(2*pi*50), Lm=(245.8954)/(2*pi*50), J=0.0088, P=4}
      mask prompts: Rs "Stator Resistance  Rs [ohms] :"; Ls "Stator Inductance Ls [Hendry] :"; Rr "Rotor Resistance Rr [ohms] :"; Lr "Rotor Inductance Lr [Hendry] :"; Lm "Mutual Inductance Lm [Hendry] :"; J "Rotor Inertia J [Kg-m2] :"; P "Number of Poles p :"
      mask help: Dynamic Modelling of Induction by using Mathematic Equations
      mask Display: fprintf('Induction\nMotor')
  Data Acquision : Subsystem
  PI Control1 : Subsystem
      mask Display: fprintf('PI\Control')
  Selector : Selector  InputPortWidth=2  IndexOptions=Index vector (dialog)  Indices=[1]  OutputSizes=1
  Subsystem : Subsystem
  Terminator : Terminator
  Terminator1 : Terminator
  VSI : Subsystem
      mask init:
      | Vdc=220;
      mask Display: fprintf('Vdc = 220 V ')
  torque : Step  Time=2  After=0  SampleTime=0
  Speedsystem : Outport
  wires:
  Data Acquision/1(is_a) -> Terminator1/1
  VSI/3(Vc) -> "1 HP , 220 V Induction Motor"/4(V_c)
  VSI/1(Va) -> "1 HP , 220 V Induction Motor"/2(V_a)
  Selector/1 -> PI Control1/2(N)
  torque/1 -> "1 HP , 220 V Induction Motor"/1(tau)
  PI Control1/1(Freq*) -> VSI/1(Freq)
  Subsystem/1("MotorSpeed ") -> PI Control1/1(N*), Data Acquision/2(speed)
  Data Acquision/2(Te(Nm)) -> Terminator/1  "Torque Te(Nm)"
  speed_ref/1 -> Subsystem/1(Speed)
  embuttom1/1 -> Subsystem/2(EmergButton1)
  embuttom2/1 -> Subsystem/3(EmergButton2)
  Data Acquision/4(wm1) -> Speedsystem/1
  Data Acquision/3(wm) -> Selector/1  "Speed( rpm)"
  VSI/2(Vb) -> "1 HP , 220 V Induction Motor"/3(V_b)
  "1 HP , 220 V Induction Motor"/1(m) -> Data Acquision/1(m)
  temp/1 -> Subsystem/4(Temperature)

== system Copy_of_TenMutantsTemplate/mutant9 ==
  note: ctrl+U to look under mask
  speed_ref : Inport
  embuttom1 : Inport  Port=2
  embuttom2 : Inport  Port=3
  temp : Inport  Port=4
  "1 HP , 220 V Induction Motor" : Subsystem  mask(Induction Motor: By SRIKANTH D){Rs=10.1, Ls=(15.81+245.8954)/(2*pi*50), Rr=9.8546, Lr=(15.81+245.8954)/(2*pi*50), Lm=(245.8954)/(2*pi*50), J=0.0088, P=4}
      mask prompts: Rs "Stator Resistance  Rs [ohms] :"; Ls "Stator Inductance Ls [Hendry] :"; Rr "Rotor Resistance Rr [ohms] :"; Lr "Rotor Inductance Lr [Hendry] :"; Lm "Mutual Inductance Lm [Hendry] :"; J "Rotor Inertia J [Kg-m2] :"; P "Number of Poles p :"
      mask help: Dynamic Modelling of Induction by using Mathematic Equations
      mask Display: fprintf('Induction\nMotor')
  Data Acquision : Subsystem
  PI Control1 : Subsystem
      mask Display: fprintf('PI\Control')
  Selector : Selector  InputPortWidth=2  IndexOptions=Index vector (dialog)  Indices=[1]  OutputSizes=1
  Subsystem : Subsystem
  Terminator : Terminator
  Terminator1 : Terminator
  VSI : Subsystem
      mask init:
      | Vdc=220;
      mask Display: fprintf('Vdc = 220 V ')
  torque : Step  Time=2  After=0  SampleTime=0
  Speedsystem : Outport
  wires:
  temp/1 -> Subsystem/4(Temperature)
  "1 HP , 220 V Induction Motor"/1(m) -> Data Acquision/1(m)
  VSI/2(Vb) -> "1 HP , 220 V Induction Motor"/3(V_b)
  Data Acquision/3(wm) -> Selector/1  "Speed( rpm)"
  Data Acquision/4(wm1) -> Speedsystem/1
  embuttom2/1 -> Subsystem/3(EmergButton2)
  embuttom1/1 -> Subsystem/2(EmergButton1)
  speed_ref/1 -> Subsystem/1(Speed)
  Data Acquision/2(Te(Nm)) -> Terminator/1  "Torque Te(Nm)"
  Subsystem/1("MotorSpeed ") -> Data Acquision/2(speed), PI Control1/1(N*)
  PI Control1/1(Freq*) -> VSI/1(Freq)
  torque/1 -> "1 HP , 220 V Induction Motor"/1(tau)
  Selector/1 -> PI Control1/2(N)
  VSI/1(Va) -> "1 HP , 220 V Induction Motor"/2(V_a)
  VSI/3(Vc) -> "1 HP , 220 V Induction Motor"/4(V_c)
  Data Acquision/1(is_a) -> Terminator1/1

== system Copy_of_TenMutantsTemplate/System/1 HP , 220 V Induction Motor ==
  tau : Inport
  V_a : Inport  Port=2
  V_b : Inport  Port=3
  V_c : Inport  Port=4
  Flux : Subsystem
  Measurements : Subsystem
  Mechanical : Subsystem
  Mux : Mux  Inputs=3
  Mux1 : Mux  Inputs=3
  abc to dq : Subsystem
  d_block : Subsystem
  dq to abc : Subsystem
  "dq to abc " : Subsystem
  q_block : Subsystem
  rad2rpm : Gain  Gain=30/pi
  m : Outport
  wires:
  Mechanical/2(omegaR) -> rad2rpm/1
  Mechanical/3(we) -> Flux/7(we)
  Flux/1(shi_ds) -> d_block/1(shi_ds), Mechanical/1(shi_ds)
  Flux/4("shi_qr ") -> q_block/2(shi_qr)
  d_block/1(i_ds) -> Mechanical/3(i_ds), Measurements/3(I_ds), dq to abc/1(I_d), Flux/3(I_ds)
  d_block/2(i_dr) -> Flux/4(I_dr), "dq to abc "/1(I_d)
  q_block/2(i_qr) -> Measurements/6(I_qr), "dq to abc "/2(I_q), Flux/6(I_qr)
  q_block/1(i_qs) -> Mechanical/4(i_qs), Measurements/4(I_dr), Measurements/5(I_qs), dq to abc/2(I_q), Flux/5(I_qs)
  Mechanical/1(Te) -> Measurements/7(Te)
  tau/1 -> Mechanical/5(tau)
  Flux/2("shi_dr ") -> d_block/2(shi_dr)
  Flux/3(shi_qs) -> q_block/1(shi_qs), Mechanical/2(shi_qs)
  abc to dq/1(V_ds) -> Flux/1(V_ds)
  abc to dq/2(V_qs) -> Flux/2(V_qs)
  V_c/1 -> abc to dq/3(Vc)
  V_b/1 -> abc to dq/2(Vb)
  V_a/1 -> abc to dq/1(Va)
  dq to abc/1(i_sa) -> Mux/1
  "dq to abc "/1(i_ra) -> Mux1/1
  dq to abc/2(i_sb) -> Mux/2
  dq to abc/3(i_sc) -> Mux/3
  "dq to abc "/3(i_rc) -> Mux1/3
  "dq to abc "/2(i_rb) -> Mux1/2
  Mux/1 -> Measurements/1(I_s)
  Mux1/1 -> Measurements/2(I_r)
  rad2rpm/1 -> Measurements/8(N)
  Measurements/1(m) -> m/1

== system Copy_of_TenMutantsTemplate/System/Data Acquision ==
  note: DONE TO HAVE AN ALLOWABLE SIMULATION TIME
  m : Inport
  speed : Inport  Port=2
  2nd-Order Filter : powerlib_extras/Control  Blocks/2nd-Order Filter  FilterType=Lowpass  Fo=120  Zeta=0.707  Initialize=off  Vac_Init=[1 45 60]  Vdc_Init=-0.5  PlotResponse=off  param1=[1 500 1]
  Bus Selector : BusSelector  OutputSignals=Mechanical.Rotor Speed in (rpm),Mechanical.Electromagnetic Torque (N*m),Stator Measurement.Stator Current i_sa (A)
  Mux : Mux  Inputs=2
  filtroPasaBajos : TransferFcn  Denominator=[1 1]
  is_a : Outport
  Te(Nm) : Outport  Port=2
  wm : Outport  Port=3
  wm1 : Outport  Port=4
  wires:
  2nd-Order Filter/1 -> Te(Nm)/1
  Bus Selector/2 -> 2nd-Order Filter/1  "<Electromagnetic Torque (N*m)>"
  m/1 -> Bus Selector/1
  Bus Selector/1 -> filtroPasaBajos/1  "<Rotor Speed in (rpm)>"
  Bus Selector/3 -> is_a/1  "<Stator Current i_sa (A)>"
  speed/1 -> Mux/2
  Mux/1 -> wm/1
  filtroPasaBajos/1 -> wm1/1, Mux/1

== system Copy_of_TenMutantsTemplate/System/PI Control1 ==
  N* : Inport
  N : Inport  Port=2
  Abs : Abs  SaturateOnIntegerOverflow=on
  Abs1 : Abs  SaturateOnIntegerOverflow=on
  Abs2 : Abs
  Compare To Constant : simulink/Logic and Bit Operations/Compare To Constant  relop=<=  const=0.1  OutDataTypeStr=uint8
  Constant : Constant  Value=0
  Divide : Product  Inputs=/*
  Integrator Limited : Integrator  LimitOutput=on  UpperSaturationLimit=30  LowerSaturationLimit=-30
  Proportional gain : Gain  Gain=0.8  SaturateOnIntegerOverflow=on  OutDataTypeStr=Inherit: Same as input  ParamDataTypeStr=Inherit: Same as input
  Rate Transition3 : RateTransition  OutPortSampleTimeOpt=Inherit
  Saturation : Saturate  UpperLimit=inf  LowerLimit=2
  Saturation2 : Saturate  UpperLimit=120  LowerLimit=0.02
  Sum1 : Sum  Inputs=|+-  SaturateOnIntegerOverflow=on  InputSameDT=on  OutDataTypeStr=Inherit: Same as first input
  Sum2 : Sum  SaturateOnIntegerOverflow=on  InputSameDT=on  OutDataTypeStr=Inherit: Same as first input
  Sum3 : Sum  Inputs=|++  SaturateOnIntegerOverflow=on  InputSameDT=on  OutDataTypeStr=Inherit: Same as first input
  Switch : Switch  Threshold=0.5
  ctrl_sat : Saturate  UpperLimit=30  LowerLimit=-30
  rpm2hz : Gain  Gain=4/120  SaturateOnIntegerOverflow=on  OutDataTypeStr=Inherit: Same as input  ParamDataTypeStr=Inherit: Same as input
  "rpm2hz  " : Gain  Gain=4/120  SaturateOnIntegerOverflow=on  OutDataTypeStr=Inherit: Same as input  ParamDataTypeStr=Inherit: Same as input
  Freq* : Outport
  wires:
  Saturation/1 -> Divide/1
  Switch/1 -> Integrator Limited/1
  Constant/1 -> Switch/3
  Compare To Constant/1 -> Switch/2
  Abs2/1 -> Divide/2
  Divide/1 -> Compare To Constant/1
  Integrator Limited/1 -> Sum2/1
  N/1 -> "rpm2hz  "/1
  Abs1/1 -> Sum1/2, Sum3/2
  Rate Transition3/1 -> Freq*/1
  Abs/1 -> Sum1/1, Saturation/1
  Sum1/1 -> Abs2/1, Switch/1, Proportional gain/1
  Saturation2/1 -> Rate Transition3/1
  "rpm2hz  "/1 -> Abs1/1
  Proportional gain/1 -> Sum2/2
  rpm2hz/1 -> Abs/1
  ctrl_sat/1 -> Sum3/1
  Sum3/1 -> Saturation2/1
  Sum2/1 -> ctrl_sat/1
  N*/1 -> rpm2hz/1

== system Copy_of_TenMutantsTemplate/System/Subsystem ==
  Speed : Inport
  EmergButton1 : Inport  Port=2
  EmergButton2 : Inport  Port=3
  Temperature : Inport  Port=4
  Compare To Constant : simulink/Logic and Bit Operations/Compare To Constant  relop=>  const=100  OutDataTypeStr=boolean
  Compare To Constant1 : simulink/Logic and Bit Operations/Compare To Constant  relop===  const=0  OutDataTypeStr=boolean
  Constant : Constant  Value=emergency_buttons
  Constant1 : Constant  Value=temperature
  Constant2 : Constant  Value=emergency_button2
  Ir_a3 : Scope
  Logical Operator : Logic  Operator=OR  AllPortsSameDT=off  OutDataTypeStr=boolean
  Logical Operator1 : Logic  AllPortsSameDT=off  OutDataTypeStr=boolean
  Logical Operator2 : Logic  AllPortsSameDT=off  OutDataTypeStr=boolean
  Logical Operator3 : Logic  AllPortsSameDT=off  OutDataTypeStr=boolean
  Speed_to_0 : Constant  Value=0
  Switch : Switch  Criteria=u2 ~= 0
  Switch1 : Switch  Criteria=u2 ~= 0
  Switch2 : Switch  Criteria=u2 ~= 0
  Transfer Fcn1 : TransferFcn  Denominator=[20 1]
  "MotorSpeed " : Outport
  wires:
  EmergButton1/1 -> Logical Operator/1
  EmergButton2/1 -> Logical Operator3/1
  Logical Operator/1 -> Logical Operator1/1
  Speed/1 -> Transfer Fcn1/1
  Switch/1 -> Switch1/3
  Speed_to_0/1 -> Switch1/1, Switch/1
  Logical Operator1/1 -> Switch/2
  Constant/1 -> Logical Operator1/2
  Temperature/1 -> Compare To Constant/1
  Compare To Constant/1 -> Logical Operator2/1
  Constant1/1 -> Logical Operator2/2
  Logical Operator2/1 -> Switch1/2
  Logical Operator3/1 -> Logical Operator/2
  Constant2/1 -> Logical Operator3/2
  Switch1/1 -> Switch2/3, Switch2/1, Compare To Constant1/1
  Switch2/1 -> Ir_a3/1, "MotorSpeed "/1
  Compare To Constant1/1 -> Switch2/2
  Transfer Fcn1/1 -> Switch/3

== system Copy_of_TenMutantsTemplate/System/VSI ==
  Freq : Inport
  Fcn : Fcn  Expr=(2*sqrt(2/3)*Vdc/3)*(2*u(1)-u(2)-u(3))
  Fcn1 : Fcn  Expr=(2*sqrt(2/3)*Vdc/3)*(2*u(2)-u(3)-u(1))
  Fcn2 : Fcn  Expr=(2*sqrt(2/3)*Vdc/3)*(2*u(3)-u(2)-u(1))
  SPWM : Subsystem
  Va : Outport
  Vb : Outport  Port=2
  Vc : Outport  Port=3
  wires:
  SPWM/1(g) -> Fcn2/1, Fcn/1, Fcn1/1
  Fcn1/1 -> Vb/1
  Fcn2/1 -> Vc/1
  Fcn/1 -> Va/1
  Freq/1 -> SPWM/1(Freq)

== system Copy_of_TenMutantsTemplate/mutant1/1 HP , 220 V Induction Motor ==
  tau : Inport
  V_a : Inport  Port=2
  V_b : Inport  Port=3
  V_c : Inport  Port=4
  Flux : Subsystem
  Measurements : Subsystem
  Mechanical : Subsystem
  Mux : Mux  Inputs=3
  Mux1 : Mux  Inputs=3
  abc to dq : Subsystem
  d_block : Subsystem
  dq to abc : Subsystem
  "dq to abc " : Subsystem
  q_block : Subsystem
  rad2rpm : Gain  Gain=30/pi
  m : Outport
  wires:
  Measurements/1(m) -> m/1
  rad2rpm/1 -> Measurements/8(N)
  Mux1/1 -> Measurements/2(I_r)
  Mux/1 -> Measurements/1(I_s)
  "dq to abc "/2(i_rb) -> Mux1/2
  "dq to abc "/3(i_rc) -> Mux1/3
  dq to abc/3(i_sc) -> Mux/3
  dq to abc/2(i_sb) -> Mux/2
  "dq to abc "/1(i_ra) -> Mux1/1
  dq to abc/1(i_sa) -> Mux/1
  V_a/1 -> abc to dq/1(Va)
  V_b/1 -> abc to dq/2(Vb)
  V_c/1 -> abc to dq/3(Vc)
  abc to dq/2(V_qs) -> Flux/2(V_qs)
  abc to dq/1(V_ds) -> Flux/1(V_ds)
  Flux/3(shi_qs) -> Mechanical/2(shi_qs), q_block/1(shi_qs)
  Flux/2("shi_dr ") -> d_block/2(shi_dr)
  tau/1 -> Mechanical/5(tau)
  Mechanical/1(Te) -> Measurements/7(Te)
  q_block/1(i_qs) -> Flux/5(I_qs), dq to abc/2(I_q), Measurements/5(I_qs), Measurements/4(I_dr), Mechanical/4(i_qs)
  q_block/2(i_qr) -> Flux/6(I_qr), "dq to abc "/2(I_q), Measurements/6(I_qr)
  d_block/2(i_dr) -> "dq to abc "/1(I_d), Flux/4(I_dr)
  d_block/1(i_ds) -> Flux/3(I_ds), dq to abc/1(I_d), Measurements/3(I_ds), Mechanical/3(i_ds)
  Flux/4("shi_qr ") -> q_block/2(shi_qr)
  Flux/1(shi_ds) -> Mechanical/1(shi_ds), d_block/1(shi_ds)
  Mechanical/3(we) -> Flux/7(we)
  Mechanical/2(omegaR) -> rad2rpm/1

== system Copy_of_TenMutantsTemplate/mutant1/Data Acquision ==
  note: DONE TO HAVE AN ALLOWABLE SIMULATION TIME
  m : Inport
  speed : Inport  Port=2
  2nd-Order Filter : powerlib_extras/Control  Blocks/2nd-Order Filter  FilterType=Lowpass  Fo=120  Zeta=0.707  Initialize=off  Vac_Init=[1 45 60]  Vdc_Init=-0.5  PlotResponse=off  param1=[1 500 1]
  Bus Selector : BusSelector  OutputSignals=Mechanical.Rotor Speed in (rpm),Mechanical.Electromagnetic Torque (N*m),Stator Measurement.Stator Current i_sa (A)
  Mux : Mux  Inputs=2
  filtroPasaBajos : TransferFcn  Denominator=[1 1]
  is_a : Outport
  Te(Nm) : Outport  Port=2
  wm : Outport  Port=3
  wm1 : Outport  Port=4
  wires:
  filtroPasaBajos/1 -> Mux/1, wm1/1
  Mux/1 -> wm/1
  speed/1 -> Mux/2
  Bus Selector/3 -> is_a/1  "<Stator Current i_sa (A)>"
  Bus Selector/1 -> filtroPasaBajos/1  "<Rotor Speed in (rpm)>"
  m/1 -> Bus Selector/1
  Bus Selector/2 -> 2nd-Order Filter/1  "<Electromagnetic Torque (N*m)>"
  2nd-Order Filter/1 -> Te(Nm)/1
